simulink model "withLoadmodel"  (R2021b)
settings: Solver=ode5  StartTime=0.0  StopTime=runT  FixedStep=dt  RelTol=1e-3
values from neighbouring files (symbols this model uses):
  Bm = bm * N * N    (= 2.601)    [noLoadInit.m]    (also in withLoadInit.m)
  den1c = [1, 2*zeta*wn, wn*wn]    [noLoadInit.m]    (also in withLoadInit.m)
  dt = 0.001    [noLoadInit.m]    (also in withLoadInit.m)
  g = -9.80665    [withLoadInit.m]
  iMax = tauMax/Kt    (= 6.13841243116)    [noLoadInit.m]    (also in withLoadInit.m = 61.3841243116)
  Jm = jm * N * N    (= 0.023968215)    [noLoadInit.m]    (also in withLoadInit.m)
  Kt = 0.1118 * N    (= 5.7018)    [noLoadInit.m]    (also in withLoadInit.m)
  linkJ = 0.25*linkM*r*r + linkM*linkL*linkL/3    (= 0.335203747348)    [withLoadInit.m]
  linkL = 1.0    (= 1)    [withLoadInit.m]
  linkM = pi*r*r*linkL*rho    (= 1.00530964915)    [withLoadInit.m]
  N = 51    [noLoadInit.m]    (also in withLoadInit.m)
  num1c = wn*wn    (= 1000000)    [noLoadInit.m]    (also in withLoadInit.m)
  tauMax = 35    [noLoadInit.m]    (also in withLoadInit.m = 350)
undefined symbols (not defined in the file or in its folder): stribeckFriction, X, Y, Z
libraries: sm_lib x6, nesl_utility x6, simulink x2
settings Model: Creator=86135  LastModifiedBy=86135

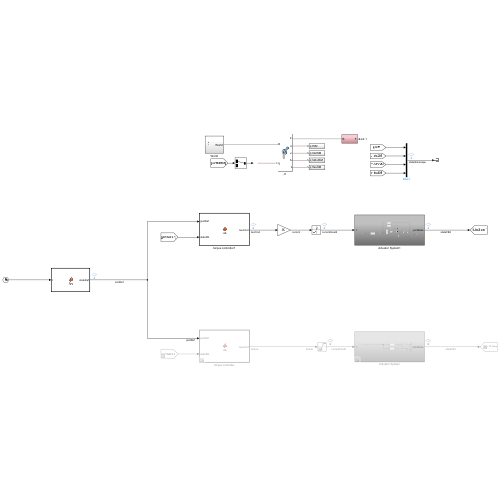
[thumbnail: Simulink's stored preview of the top-level diagram]
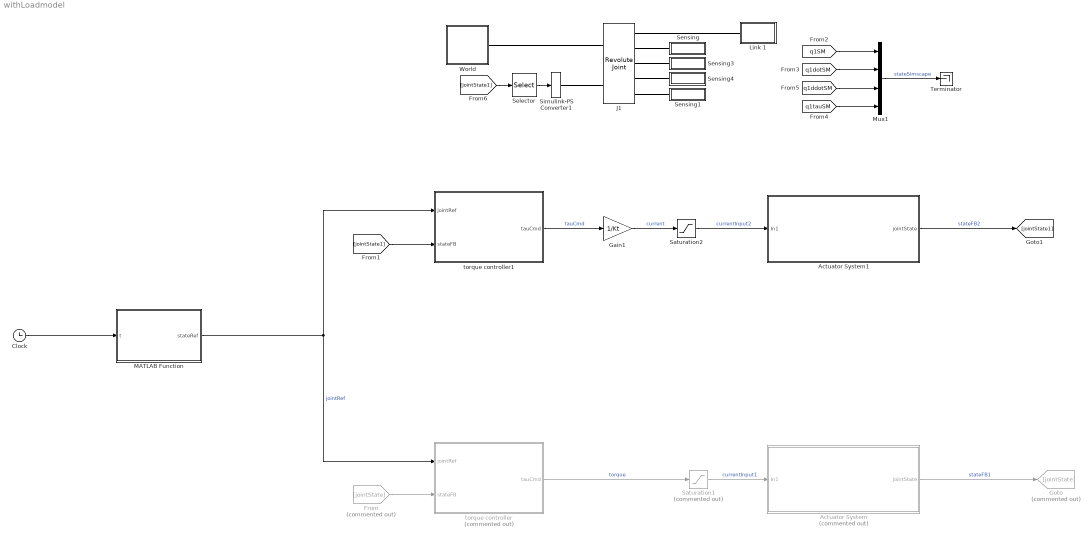
== system withLoadmodel ==
  Actuator System : Subsystem  Commented=on
  Actuator System1 : Subsystem
  Clock : Clock
  From : From  Commented=on  GotoTag=jointState
  Gain1 : Gain  Gain=1/Kt
  Goto : Goto  Commented=on  GotoTag=jointState
  J1 : sm_lib/Joints/Revolute Joint  JointMode=Normal  SenseConstraintForce=off  SenseConstraintForceX=off  SenseConstraintForceY=off  SenseConstraintForceZ=off  SenseConstraintTorque=off  SenseConstraintTorqueX=off  SenseConstraintTorqueY=off  SenseConstraintTorqueZ=off  SenseTotalForce=off  SenseTotalForceX=off  SenseTotalForceY=off  SenseTotalForceZ=off  SenseTotalTorque=off  SenseTotalTorqueX=off  SenseTotalTorqueY=off  SenseTotalTorqueZ=off  CompositeWrenchDir=FollowerOnBase  CompositeWrenchFrame=BaseFrame  EquilibriumPosition=0  EquilibriumPositionUnits=rad  SpringStiffness=0  SpringStiffnessUnits=N*m/rad  DampingCoefficient=0.0  DampingCoefficientUnits=N*m/(rad/s)  TorqueActuationMode=ComputedTorque  MotionActuationMode=InputMotion  SensePosition=on  SenseVelocity=on  SenseAcceleration=on  SenseTorqueForce=on  SenseLowerLimitTorqueForce=off  SenseUpperLimitTorqueForce=off  LowerLimitSpecify=off  LowerLimitBound=-90  LowerLimitBoundUnits=deg  LowerLimitStiffness=1e4  LowerLimitStiffnessUnits=N*m/deg  LowerLimitDamping=10  LowerLimitDampingUnits=N*m/(deg/s)  LowerLimitTransitionRegionWidth=0.1  LowerLimitTransitionRegionWidthUnits=deg  UpperLimitSpecify=off  UpperLimitBound=90  UpperLimitBoundUnits=deg  UpperLimitStiffness=1e4  UpperLimitStiffnessUnits=N*m/deg  UpperLimitDamping=10  UpperLimitDampingUnits=N*m/(deg/s)  UpperLimitTransitionRegionWidth=0.1  UpperLimitTransitionRegionWidthUnits=deg  PositionTargetSpecify=off  PositionTargetPriority=Low  PositionTargetValue=0  PositionTargetValueUnits=rad  VelocityTargetSpecify=off  VelocityTargetPriority=High  VelocityTargetValue=0  VelocityTargetValueUnits=rad/s
  Link 1 : Subsystem  Tag=CustomStyle
  MATLAB Function : MATLAB Function  TreatAsAtomicUnit=on
  Mux1 : Mux
  Saturation1 : Saturate  Commented=on  UpperLimit=tauMax  LowerLimit=-tauMax
  Saturation2 : Saturate  UpperLimit=iMax  LowerLimit=-iMax
  Selector : Selector  InputPortWidth=2  IndexOptions=Index vector (dialog)  Indices=[1]  OutputSizes=1
  Sensing : Subsystem
  Sensing1 : Subsystem
  Sensing3 : Subsystem
  Sensing4 : Subsystem
  Simulink-PS Converter1 : nesl_utility/Simulink-PS Converter  PhysicalDomain=network_engine_domain  SubClassName=ps_input  LeftPortType=input  RightPortType=output  PseudoPeriodic=off  Frequencies=[]  NoiseDistribution=none  NoiseParameters=[]  Unit=1  AffineConversion=off  FilteringAndDerivatives=filter  SimscapeFilterOrder=2  InputFilterTimeConstant=dt  UdotUserProvided=2
      settings: SourceProductBaseCode=PW,SS
  Terminator : Terminator
  World : Subsystem
  torque controller : MATLAB Function  Commented=on  TreatAsAtomicUnit=on
  torque controller1 : MATLAB Function  TreatAsAtomicUnit=on
  wires:
  torque controller/1(tauCmd) -> Saturation1/1  "torque"
  Saturation1/1 -> Actuator System/1(In1)  "currentInput1"
  Actuator System/1(jointState) -> Goto/1  "stateFB1"
  From/1 -> torque controller/2(stateFB)
  MATLAB Function/1(stateRef) -> torque controller/1(jointRef), torque controller1/1(jointRef)  "jointRef"
  Actuator System1/1(jointState) -> [jointState1]  "stateFB2"
  [jointState1] -> torque controller1/2(stateFB)
  torque controller1/1(tauCmd) -> Gain1/1  "tauCmd"
  Gain1/1 -> Saturation2/1  "current"
  Saturation2/1 -> Actuator System1/1(In1)  "currentInput2"
  [q1ddotSM] -> Mux1/3
  Mux1/1 -> Terminator/1  "stateSimscape"
  [q1SM] -> Mux1/1
  [q1dotSM] -> Mux1/2
  [q1tauSM] -> Mux1/4
  [jointState1] -> Selector/1
  Selector/1 -> Simulink-PS Converter1/1
  Clock/1 -> MATLAB Function/1(t)
  connections:
  Sensing3/LConn1 -- J1/RConn3
  Link 1/RConn1 -- J1/RConn1
  J1/LConn1 -- World/RConn1
  Sensing/LConn1 -- J1/RConn2
  Sensing4/LConn1 -- J1/RConn4
  Sensing1/LConn1 -- J1/RConn5
  Simulink-PS Converter1/RConn1 -- J1/LConn2

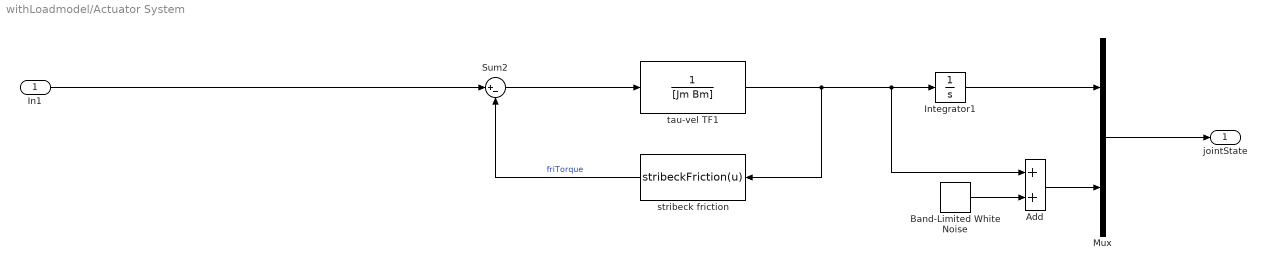
== system withLoadmodel/Actuator System ==
  In1 : Inport
  Add : Sum
  Band-Limited White Noise : simulink/Sources/Band-Limited White Noise  Cov=[0.00002]  Ts=0.001  seed=noiseSeedIndex
  Integrator1 : Integrator
  Mux : Mux  Inputs=2
  Sum2 : Sum  Inputs=|+-
  stribeck friction : MATLABFcn  MATLABFcn=stribeckFriction(u)
  tau-vel TF1 : TransferFcn  Denominator=[Jm Bm]
  jointState : Outport
  wires:
  tau-vel TF1/1 -> stribeck friction/1, Add/1, Integrator1/1
  stribeck friction/1 -> Sum2/2  "friTorque"
  Sum2/1 -> tau-vel TF1/1
  In1/1 -> Sum2/1
  Integrator1/1 -> Mux/1
  Add/1 -> Mux/2
  Mux/1 -> jointState/1
  Band-Limited White Noise/1 -> Add/2

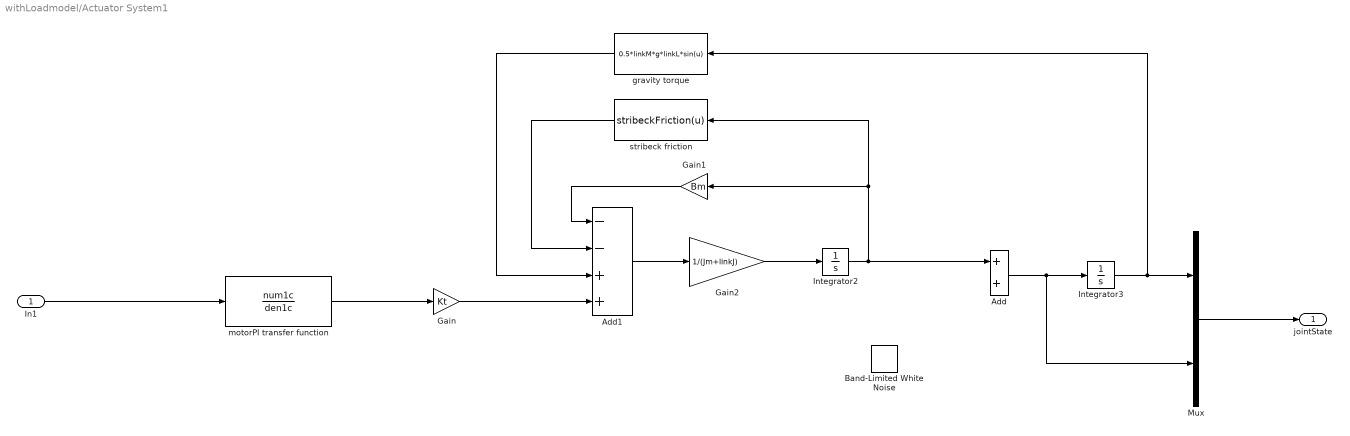
== system withLoadmodel/Actuator System1 ==
  In1 : Inport
  Add : Sum
  Add1 : Sum  Inputs=--++
  Band-Limited White Noise : simulink/Sources/Band-Limited White Noise  Cov=[0.00002]  Ts=0.001  seed=noiseSeedIndex
  Gain : Gain  Gain=Kt
  Gain1 : Gain  Gain=Bm
  Gain2 : Gain  Gain=1/(Jm+linkJ)
  Integrator2 : Integrator
  Integrator3 : Integrator
  Mux : Mux  Inputs=2
  gravity torque : MATLABFcn  MATLABFcn=0.5*linkM*g*linkL*sin(u)
  motorPI transfer function : TransferFcn  Numerator=num1c  Denominator=den1c
  stribeck friction : MATLABFcn  MATLABFcn=stribeckFriction(u)
  jointState : Outport
  wires:
  Gain1/1 -> Add1/1
  Add1/1 -> Gain2/1
  In1/1 -> motorPI transfer function/1
  Integrator2/1 -> Add/1, stribeck friction/1, Gain1/1
  Gain2/1 -> Integrator2/1
  Mux/1 -> jointState/1
  Add/1 -> Mux/2, Integrator3/1
  stribeck friction/1 -> Add1/2
  Integrator3/1 -> gravity torque/1, Mux/1
  motorPI transfer function/1 -> Gain/1
  Gain/1 -> Add1/4
  gravity torque/1 -> Add1/3

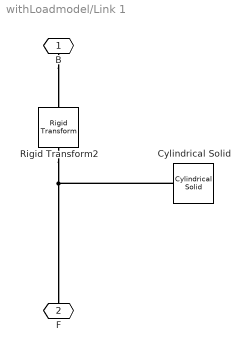
== system withLoadmodel/Link 1 ==
  Cylindrical Solid : sm_lib/Body Elements/Cylindrical Solid  GraphicAmbientColor=[0.15 0.15 0.15 1.0]  BasedOnType=Density  CenterOfMass=[0 0 0]  CenterOfMassUnits=m  GraphicDiffuseColor=[0.0 0.0 1.0]  CylinderLength=1  CylinderLengthUnits=m  CylinderRadius=0.02  CylinderRadiusUnits=m  Density=rho  DensityUnits=kg/m^3  DoExposeReferenceFrame=on  GraphicEmissiveColor=[0.0 0.0 0.0 1.0]  ExportEntireGeometry=off  SerializedFrames=<Frames><Frame><Id>Frame1</Id><Value><Name>F1</Name><Origin><Source>GeometricFeature</Source><FeatureName>top curve</FeatureName></Origin><PrimaryAxis><DefinedDirection>+Z</DefinedDirection><Source>ReferenceFrame</Source><SourceDirection>+Z</SourceDirection><FeatureName></FeatureName></PrimaryAxis><SecondaryAxis><DefinedDirection>+X</DefinedDirection><Source>ReferenceFrame</Source><SourceDirection>+X</SourceDirection><FeatureName></FeatureName></SecondaryAxis></Value></Frame></Frames>  MarkerShape=Sphere  MarkerSize=10  GraphicType=FromGeometry  InertiaType=Custom  Mass=linkM  MassUnits=kg  MomentsOfInertia=linkMOI  MomentsOfInertiaUnits=kg*m^2  GraphicOpacity=1.0  ProductsOfInertia=[0 0 0]  ProductsOfInertiaUnits=kg*m^2  GraphicShininess=75  GraphicSpecularColor=[0.5 0.5 0.5 1.0]  GraphicVisPropType=SimpleVisualProperties
  Rigid Transform2 : sm_lib/Frames and Transforms/Rigid Transform  TranslationMethod=None  TranslationStandardOffset=0  TranslationLengthUnit=m  TranslationStandardAxis=+Z  TranslationCartesianOffset=[0 0 0]  TranslationROffset=0  TranslationROffsetUnits=m  TranslationZOffset=0  TranslationZOffsetUnits=m  TranslationThetaOffset=0  TranslationThetaOffsetUnits=deg  RotationMethod=StandardAxis  RotationAngleUnits=deg  RotationStandardAxis=+Y  RotationAngle=-90  RotationArbitraryAxis=[0 0 1]  FollAlignAxisA=+X  BaseAlignAxisA=+Y  FollAlignAxisB=+Y  BaseAlignAxisB=+Z  RotationSequenceAxes=FollowerAxes  RotationSequence=XYX  RotationSequenceAngles=[0 0 0]  RotationSequenceAnglesUnits=deg  RotationMatrix=[1 0 0; 0 1 0; 0 0 1]
  B : PMIOPort  Side=Right
  F : PMIOPort  Port=2  Side=Left
  connections:
  B/RConn1 -- Rigid Transform2/LConn1
  Rigid Transform2/RConn1 -- Cylindrical Solid/LConn1 -- F/RConn1

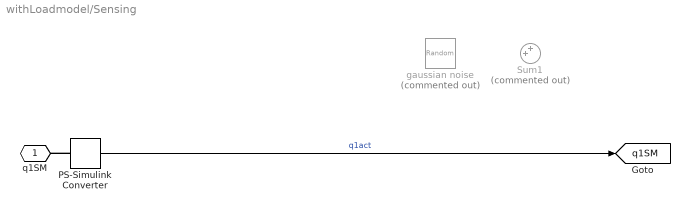
== system withLoadmodel/Sensing ==
  PS-Simulink Converter : nesl_utility/PS-Simulink Converter  PhysicalDomain=network_engine_domain  SubClassName=ps_output  LeftPortType=input  RightPortType=output  PseudoPeriodic=off  Frequencies=[]  Unit=rad  AffineConversion=off
      settings: SourceProductBaseCode=PW,SS
  Sum1 : Sum  Commented=on  Inputs=++|
  gaussian noise : RandomNumber  Commented=on  Variance=0.0001  Seed=41  SampleTime=dt
  q1SM : PMIOPort  Side=Left
  tag scope: q1SM=global
  wires:
  PS-Simulink Converter/1 -> [q1SM]  "q1act"
  connections:
  PS-Simulink Converter/LConn1 -- q1SM/RConn1

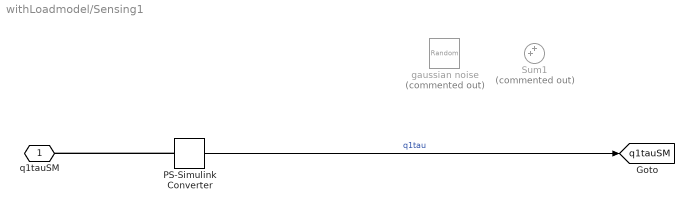
== system withLoadmodel/Sensing1 ==
  PS-Simulink Converter : nesl_utility/PS-Simulink Converter  PhysicalDomain=network_engine_domain  SubClassName=ps_output  LeftPortType=input  RightPortType=output  PseudoPeriodic=off  Frequencies=[]  Unit=N*m  AffineConversion=off
      settings: SourceProductBaseCode=PW,SS
  Sum1 : Sum  Commented=on  Inputs=++|
  gaussian noise : RandomNumber  Commented=on  Variance=0.0001  Seed=41  SampleTime=dt
  q1tauSM : PMIOPort  Side=Left
  tag scope: q1tauSM=global
  wires:
  PS-Simulink Converter/1 -> [q1tauSM]  "q1tau"
  connections:
  PS-Simulink Converter/LConn1 -- q1tauSM/RConn1

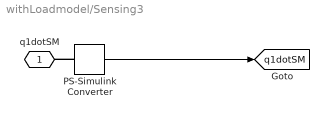
== system withLoadmodel/Sensing3 ==
  PS-Simulink Converter : nesl_utility/PS-Simulink Converter  PhysicalDomain=network_engine_domain  SubClassName=ps_output  LeftPortType=input  RightPortType=output  PseudoPeriodic=off  Frequencies=[]  Unit=1  AffineConversion=off
      settings: SourceProductBaseCode=PW,SS
  q1dotSM : PMIOPort  Side=Left
  tag scope: q1dotSM=global
  wires:
  PS-Simulink Converter/1 -> [q1dotSM]
  connections:
  PS-Simulink Converter/LConn1 -- q1dotSM/RConn1

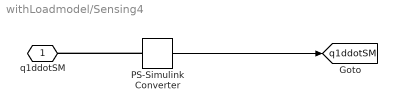
== system withLoadmodel/Sensing4 ==
  PS-Simulink Converter : nesl_utility/PS-Simulink Converter  PhysicalDomain=network_engine_domain  SubClassName=ps_output  LeftPortType=input  RightPortType=output  PseudoPeriodic=off  Frequencies=[]  Unit=1  AffineConversion=off
      settings: SourceProductBaseCode=PW,SS
  q1ddotSM : PMIOPort  Side=Left
  tag scope: q1ddotSM=global
  wires:
  PS-Simulink Converter/1 -> [q1ddotSM]
  connections:
  PS-Simulink Converter/LConn1 -- q1ddotSM/RConn1

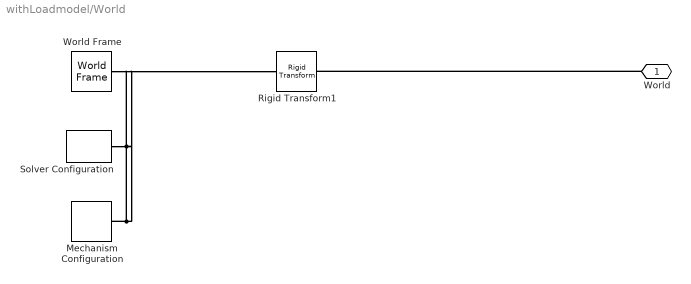
== system withLoadmodel/World ==
  Mechanism Configuration : sm_lib/Utilities/Mechanism Configuration  UniformGravity=Constant  GravityVector=simPara.gravity  GravityUnits=m/s^2  LinearizationDelta=0.001  JointModeTransitionNonlinearIterations=2
  Rigid Transform1 : sm_lib/Frames and Transforms/Rigid Transform  TranslationMethod=None  TranslationStandardOffset=0  TranslationLengthUnit=m  TranslationStandardAxis=+Z  TranslationCartesianOffset=[0 0 0]  TranslationROffset=0  TranslationROffsetUnits=m  TranslationZOffset=0  TranslationZOffsetUnits=m  TranslationThetaOffset=0  TranslationThetaOffsetUnits=deg  RotationMethod=StandardAxis  RotationAngleUnits=deg  RotationStandardAxis=+Y  RotationAngle=90  RotationArbitraryAxis=[0 0 1]  FollAlignAxisA=+X  BaseAlignAxisA=+Y  FollAlignAxisB=+Y  BaseAlignAxisB=+Z  RotationSequenceAxes=FollowerAxes  RotationSequence=XYX  RotationSequenceAngles=[0 0 0]  RotationSequenceAnglesUnits=deg  RotationMatrix=[1 0 0; 0 1 0; 0 0 1]
  Solver Configuration : nesl_utility/Solver Configuration  PhysicalDomain=network_engine_domain  SubClassName=solver  LeftPortType=input  RightPortType=generic  Tones=[]  Harmonics=[]  SimulateNoise=off  Profile=off  UseLocalSampling=off  EnableSwitchedLinearOptims=on  FrequencyDomain=off  UseCCode=off  RelTol=0.001  AbsTol=1e-06  MinStep=1e-09  ToWorkspace=off  RevertToSquareIcSolve=off  NumHomotopyIterations=100  PhasorMode=off  PhasorModeNumHarmonics=1  DoDC=off  ResidualTolerance=1e-9  UseLocalSolver=off  LocalSolverChoice=NE_BACKWARD_EULER_ADVANCER  LocalSolverSampleTime=.001  DoFixedCost=off  MaxNonlinIter=3  MaxModeIter=2  ComputeImpulses=off  ImpulseIterations=2  LinearAlgebra=Sparse  EquationFormulation=NE_TIME_EF  DelaysMemoryBudget=1024  AutomaticFiltering=on  FilteringTimeConstant=0.001  PartitionStorageMethod=AS_NEEDED  PartitionMemoryBudget=1024  PartitionMethod=FAST
      settings: SourceProductBaseCode=PW,SS
  World Frame : sm_lib/Frames and Transforms/World Frame
  World : PMIOPort  Side=Right
  connections:
  Mechanism Configuration/RConn1 -- Rigid Transform1/LConn1 -- World Frame/RConn1 -- Solver Configuration/RConn1
  World/RConn1 -- Rigid Transform1/RConn1

== matlab function withLoadmodel/torque controller1 ==
  data: jointRef input; tauCmd output; stateFB input; simPara parameter
function tauCmd = fcn(jointRef, stateFB, simPara)

qRef    = jointRef(1);
qdRef   = jointRef(2);
qddRef  = jointRef(3);
qFB     = stateFB(1);
qdFB    = stateFB(2);

Jm = simPara.Jm;
Bm = simPara.Bm;
kp = simPara.kp;
kd = simPara.kd;
g = simPara.gravity(3);
linkL = simPara.linkL;
linkM = simPara.linkM;
linkJ = simPara.linkJ;

friTorqueFFD = stribeckFriction(qdFB);
gravityTorque = - 0.5 * linkM * g * linkL * sin(qRef);

qError = qRef - qFB;
qdError = qdRef - qdFB;

feedbackTorque = kp * qError + kd * qdError;
feedforwardTorque = friTorqueFFD + (Jm+linkJ) * qddRef + Bm * qdRef + gravityTorque;

tauCmd = feedbackTorque + feedforwardTorque;

== matlab function withLoadmodel/torque controller ==
  data: jointRef input; tauCmd output; stateFB input; simPara parameter
function tauCmd = fcn(jointRef, stateFB, simPara)

qRef    = jointRef(1);
qdRef   = jointRef(2);
qddRef  = jointRef(3);
qFB     = stateFB(1);
qdFB    = stateFB(2);

Jm = simPara.Jm;
Bm = simPara.Bm;
kp = simPara.kp;
kd = simPara.kd;

friTorqueFFD = stribeckFriction(qdFB);

qError = qRef - qFB;
qdError = qdRef - qdFB;

feedbackTorque = kp * qError + kd * qdError;
feedforwardTorque = friTorqueFFD + Jm * qddRef + Bm * qdRef;
tauCmd = feedbackTorque + feedforwardTorque;
% tauCmd = feedforwardTorque;

== matlab function withLoadmodel/MATLAB Function ==
  data: t input; stateRef output
function stateRef = fcn(t)

A = pi/2;
T = 2;
k = 2*pi/T;

q   = +A * sin(k*t);
qd  = +A * cos(k*t) * k;
qdd = -A * sin(k*t) * k * k;

stateRef = [q;qd;qdd];
